simulink model "A3_S28"  (R2015a)
settings: Solver=ode45  StartTime=0.0  StopTime=300  RelTol=1e-3
settings Model: Creator=James  LastModifiedBy=James

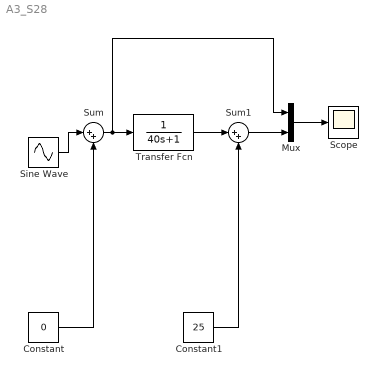
== system A3_S28 ==
  Constant : Constant  Value=0
  Constant1 : Constant  Value=25
  Mux : Mux  Inputs=2
  Scope : Scope
  Sine Wave : Sin  Amplitude=10  Frequency=6.28/24  Phase=-6.28*8/24  SampleTime=0
  Sum : Sum  Inputs=|++
  Sum1 : Sum  Inputs=|++
  Transfer Fcn : TransferFcn  Denominator=[40 1]
  wires:
  Sine Wave/1 -> Sum/1
  Sum/1 -> Mux/1, Transfer Fcn/1
  Constant/1 -> Sum/2
  Mux/1 -> Scope/1
  Transfer Fcn/1 -> Sum1/1
  Constant1/1 -> Sum1/2
  Sum1/1 -> Mux/2
